simulink model "FocESMOGenerator"  (R2024a)
settings: Solver=FixedStepDiscrete  StartTime=0.0  StopTime=5  FixedStep=0.00005  RelTol=1e-3
values from neighbouring files (symbols this model uses):
  Ld = 5.135e-05    [ASMO_HFI_Generator.mat]
  Max_Current = 10    [ASMO_HFI_Generator.mat]
  Pole = 10    [ASMO_HFI_Generator.mat]
  Rs = 0.082    [ASMO_HFI_Generator.mat]
  Switch_Speed = 500    [ASMO_HFI_Generator.mat]
  UdInjectVal = 2.5    [ASMO_HFI_Generator.mat]
undefined symbols (not defined in the file or in its folder): DiscIntNeverNeededParam
libraries: slpidlib x5
(part 2 of 2)

== system FocESMOGenerator/FocSensorLess_ASMO/SVPWM/InvClark ==
  Ualpha : Inport  OutDataTypeStr=single
  Ubeta : Inport  Port=2  OutDataTypeStr=single
  Gain : Gain  Gain=-1/2  OutDataTypeStr=single
  Gain1 : Gain  Gain=sqrt(3)/2  OutDataTypeStr=single
  Sum : Sum  Inputs=|++  OutDataTypeStr=single
  Sum1 : Sum  Inputs=-+|  OutDataTypeStr=single
  Ua : Outport  OutDataTypeStr=single
  Ub : Outport  Port=2  OutDataTypeStr=single
  Uc : Outport  Port=3  OutDataTypeStr=single
  wires:
  Ualpha/1 -> Gain/1, Ua/1
  Ubeta/1 -> Gain1/1
  Gain/1 -> Sum1/2, Sum/1
  Sum/1 -> Ub/1
  Gain1/1 -> Sum/2, Sum1/1
  Sum1/1 -> Uc/1

== system FocESMOGenerator/FocSensorLess_ASMO/SVPWM/ei_t ==
  Uabc : Inport  OutDataTypeStr=single
  Demux : Demux  Outputs=3
  Gain : Gain  Gain=-1/2  OutDataTypeStr=single
  Min : MinMax  Inputs=3  OutDataTypeStr=single
  Min1 : MinMax  Function=max  Inputs=3  OutDataTypeStr=single
  Sum : Sum  Inputs=|++  OutDataTypeStr=single
  ei_t : Outport  OutDataTypeStr=single
  wires:
  Min/1 -> Sum/1
  Sum/1 -> Gain/1
  Min1/1 -> Sum/2
  Gain/1 -> ei_t/1
  Uabc/1 -> Demux/1
  Demux/1 -> Min1/1, Min/1
  Demux/2 -> Min/2, Min1/2
  Demux/3 -> Min1/3, Min/3

== system FocESMOGenerator/FocSensorLess_ASMO/HFI_Inject/Subsystem/If Action Subsystem ==
  In1 : Inport
  Action Port : ActionPort  ActionPortLabel=if(u1 == 1)
  Output : Outport
  wires:
  In1/1 -> Output/1

== system FocESMOGenerator/FocSensorLess_ASMO/HFI_Inject/Subsystem/If Action Subsystem1 ==
  In1 : Inport
  Action Port : ActionPort  ActionPortLabel=elseif(u1 == 0)
  Output : Outport
  wires:
  In1/1 -> Output/1

== system FocESMOGenerator/FocSensorLess_ASMO/HFI_Inject/Subsystem/If Action Subsystem2 ==
  In1 : Inport
  Action Port : ActionPort  ActionPortLabel=else
  Output : Outport
  wires:
  In1/1 -> Output/1
